simulink model "BoostPFC"  (R2024b)
settings: Solver=FixedStepAuto  StartTime=0.0  StopTime=3  FixedStep=Ts  RelTol=1e-3
PreLoadFcn:
  | BoostPFCData
values from neighbouring files (symbols this model uses):
  Delta = 1-V_I/V_O    (= 0.4)    [DCDCTuning.m]
  f_sw = 50e3    (= 50000)    [DCDCTuning.m]
  Ki_v = X_pid(2)    [DCDCTuning.m]
  Kp_v = X_pid(1)    [DCDCTuning.m]
  R = 40    [DCDCTuning.m]
  Ts = 1/(30*f_sw)    (= 6.66666666667e-07)    [DCDCTuning.m]
  Tsc = 1/(f_sw)    (= 2e-05)    [DCDCTuning.m]
  V_I = 24    [DCDCTuning.m]
undefined symbols (not defined in the file or in its folder): Ki_i, Kp_i
libraries: fl_lib x14, nesl_utility x7, eePwmGenerator x1, ee_lib x1, spsPowerLib x1
CloseFcn:
  | try,close(h1_ee_BoostPFC),end
  | clear h1_BoostPFC
  | 
  | clear simlog_BoostPFC
  | clear logsout_BoostPFC
Description:
  | Power Factor Correction for CCM Boost Converter
  | 
  | %
settings Model: Creator=The MathWorks, Inc.  LastModifiedBy=Will
settings SolverCC: AlgebraicLoopSolver=TrustRegion  MaxZcPerStep=1
settings DataIOCC: FinalStateName=xTransients  InitialState=xTransients  SaveOperatingPoint=on  SaveOutput=off  SignalLogging=off  DSMLogging=off  SaveTime=off  ReturnWorkspaceOutputs=off
settings OptimizationCC: ReuseModelBlockBuffer=off  LifeSpan=inf
settings DebuggingCC: UnconnectedInputMsg=warning  UnconnectedOutputMsg=warning  UnconnectedLineMsg=warning  SFUnexpectedBacktrackingDiag=warning  SFNoUnconditionalDefaultTransitionDiag=warning  SFExecutionAtInitializationDiag=none  ArithmeticOperatorsInVariantConditions=warning
settings ModelReferenceCC: EnableRefExpFcnMdlSchedulingChecks=on
settings SFSimCC: SimUseLocalCustomCode=off  CustomCodeUndefinedFunction=UseInterfaceOnly
settings RTWCC: RTWUseLocalCustomCode=off  GPUComputeCapability=3.5  DLArmComputeVersion=19.05
settings CodeAppCC: StateflowObjectComments=on
settings GRTTargetCC: TargetLangStandard=C89/C90 (ANSI)
settings ConfigComp: CovMetricSettings=dw  CovSaveCumulativeToWorkspaceVar=on  CovSaveSingleToWorkspaceVar=on  CovExternalEMLEnable=off
settings SimscapeCC: SimscapeNormalizeSystem=off  SimscapeLogType=local  SimscapeLogName=simlog_BoostPFC  SimscapeLogLimitData=off

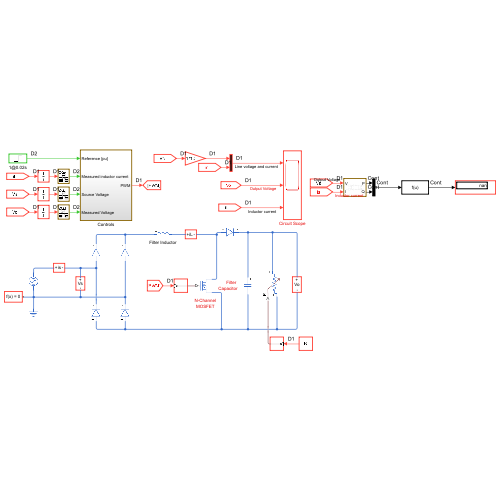
[thumbnail: Simulink's stored preview of the top-level diagram]
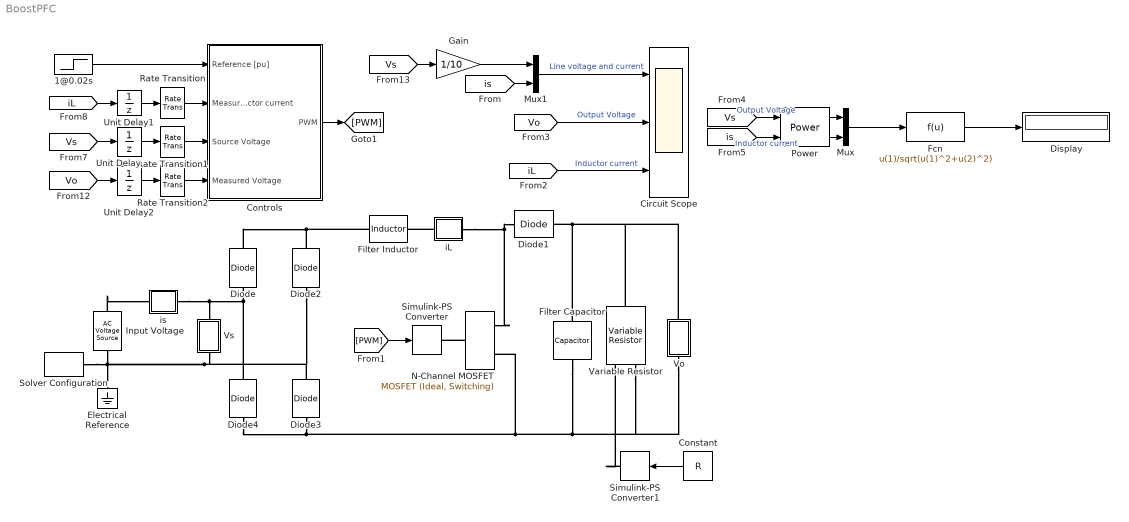
== system BoostPFC ==
  1@0.02s : Step  Time=0.02  After=40  SampleTime=Tsc
  Circuit Scope : Scope  NumInputPorts=3
  Constant : Constant  Value=R  SampleTime=Ts
  Controls : Subsystem
  Diode{,2..4} (4 alike) : fl_lib/Electrical/Electrical Elements/Diode  Vf=0.6 V  Ron=0.3 Ohm  Goff=1e-8 1/Ohm  i_specify=off  i_priority=None  i=0 A  i_nominal_specify=off  i_nominal_value=1  i_nominal_unit=A  v_specify=off  v_priority=None  v=0 V  v_nominal_specify=off  v_nominal_value=1  v_nominal_unit=V
  Diode1 : fl_lib/Electrical/Electrical Elements/Diode  Vf=0.55 V  Ron=0.36 Ohm  Goff=1e-8 1/Ohm  i_specify=off  i_priority=None  i=0 A  i_nominal_specify=off  i_nominal_value=1  i_nominal_unit=A  v_specify=off  v_priority=None  v=0 V  v_nominal_specify=off  v_nominal_value=1  v_nominal_unit=V
  Display : Display
  Electrical Reference : fl_lib/Electrical/Electrical Elements/Electrical Reference
  Fcn : Fcn  Expr=u(1)/sqrt(u(1)^2+u(2)^2)
  Filter Capacitor : fl_lib/Electrical/Electrical Elements/Capacitor  c=Cap F  r=r_C Ohm  g=0 1/Ohm  i_specify=off  i_priority=None  i=0 A  i_nominal_specify=off  i_nominal_value=1  i_nominal_unit=A  v_specify=off  v_priority=None  v=0 V  v_nominal_specify=off  v_nominal_value=1  v_nominal_unit=V  vc_specify=off  vc_priority=High  vc=0 V  vc_nominal_specify=off  vc_nominal_value=1  vc_nominal_unit=V
  Filter Inductor : fl_lib/Electrical/Electrical Elements/Inductor  l=L H  r=r_L Ohm  g=1e-9 1/Ohm  i_specify=off  i_priority=None  i=20 A  i_nominal_specify=off  i_nominal_value=1  i_nominal_unit=A  v_specify=off  v_priority=None  v=0 V  v_nominal_specify=off  v_nominal_value=1  v_nominal_unit=V  i_L_specify=off  i_L_priority=High  i_L=0 A  i_L_nominal_specify=off  i_L_nominal_value=1  i_L_nominal_unit=A
      settings: LogSimulationData=on
  Gain : Gain  Gain=1/10
  Input Voltage : fl_lib/Electrical/Electrical Sources/AC Voltage Source  amp=V_I*sqrt(2) V  shift=0 deg  frequency=f_line Hz
  Mux : Mux  Inputs=2
  Mux1 : Mux  Inputs=2
  N-Channel MOSFET : ee_lib/Semiconductors & Converters/MOSFET (Ideal, Switching)  port_option=ee.enum.controlport.ps  Rds=0.005 Ohm  Goff=1e-6 1/Ohm  Vth=0.5 V  diode_param=2  diode_Vf=0.88 V  diode_Ron=0.001 Ohm  diode_Goff=1e-5 1/Ohm  diode_C=5e-8 F  diode_iRM=-235 A  diode_iF=300 A  diode_idot=-50 A/us  diode_trr_param=1  diode_trr_factor=3  diode_trr=15 us  diode_Qrr=1.5e+3 s*uA  ids_specify=off  ids_priority=None  ids=0 A  ids_nominal_specify=off  ids_nominal_value=1  ids_nominal_unit=A  vds_specify=off  vds_priority=None  vds=0 V  vds_nominal_specify=off  vds_nominal_value=1  vds_nominal_unit=V  vgs_specify=off  vgs_priority=None  vgs=0 V  vgs_nominal_specify=off  vgs_nominal_value=1  vgs_nominal_unit=V  thermal_loss_option=ee.enum.converters.thermalLossOption.constantvalues  Von_data=[0, 1.8, 3.2, 6, 10, 16; 0, 2, 5.5, 9.5, 15, 25] V  Tj=[298.15, 448.15] K  Iout_data=[0, 20, 40, 60, 80, 100] A  Eon_data=[0, 55.04, 124.57, 235.53, 362.12; 0, 71.25, 161.25, 304.88, 468.75] * 1e-6 J  Eoff_data=[0, 18, 30, 56.1, 76.5; 0, 22.5, 37.5, 70.13, 95.63] * 1e-6 J  Eon_data_3D=[zeros(2, 5, 3)] J  Eoff_data_3D=[zeros(2, 5, 3)] J  Tj_loss=[298.15, 448.15] K  Iout_data_loss=[0, 10, 20, 30, 40] A  tabulateWithVds=false  Vds_loss=[0, 150, 300] V  Eon_scalar=22.86e-3 J  Eoff_scalar=17.14e-3 J  Voff=300 V  Iout_scalar=600 A  useCurrentFromPreviousCycle=false  useVoltageFromPreviousCycle=false  diodeModelType=ee.enum.converters.diodeModelType.pwl  diodeTableType=ee.enum.diode.tableType.IfMat  diode_ReverseIVType=ee.enum.diode.diodeReverseIV.constant  diode_IfMat=[.07, .12, .19, 1.75, 4.24, 7.32, 11.2; .16, .3, .72, 2.14, 4.02, 6.35, 9.12] A  diode_VfMat=[.9, 1.15, 1.25, 1.5, 1.75, 2.17, 2.6, 2.85; .58, .68, .75, 1.1, 1.38, 1.77, 2.27, 2.7] V  diode_TjVec=[25, 125] degC  diode_VfVec=[.5, .7, .9, 1.3, 1.7, 2.1, 2.5] V  diode_IfVec=[.1, .2, .5, 1, 2, 4, 7, 10] A  diode_IrMat=[1e-06, 2e-06, 5e-06, 1e-05, 2.5e-05, 5e-05, .0001; 2e-06, 5e-06, 1e-05, 4e-05, 8e-05, .0002, .0005] A  diode_VrMat=[10, 100, 200, 250, 300, 325, 350; 10, 70, 160, 220, 270, 300, 320] V  diode_VrVec=[10, 20, 40, 50, 70, 80, 100] V  diode_IrVec=[1e-06, 2e-06, 5e-06, 1e-05, 2e-05, 5e-05, .0001] A  diode_Vr=-600 V  diode_Ls=150 nH  diode_Erec=0.03 J  diode_rec_loss_model=ee.enum.diode.reverseRecoveryModel.fixed  diode_ErecVal=0 J  diode_scaleWithIandV=true  diode_ErecMat=zeros(2, 3) J  diode_TjrecVec=[298.15, 398.15] K  diode_IfrecVec=[.1, 1, 10] A  diode_IrecVal=10 A  diode_VrecVal=10 V  diode_tFilter=1 / 1000 / 100 s  separateThermalPortForDiode=false  thermal_network_parameterization=ee.enum.thermalNetworkTopology.external  Rth=[.03, .2] K/W  Rth_Cauer=[.03, .1, .2] K/W  Rth_Foster=[.03, .2] K/W  thermal_mass_parameterization=ee.enum.thermalNetwork.timeconstant  thermal_mass=[3, 25] J/K  thermal_mass_Cauer=[3, 10, 25] J/K  thermal_mass_Foster=[33, 50] J/K  thermal_time_constant=[.1, 5] s  thermal_time_constant_Cauer=[.1, 1, 5] s  thermal_time_constant_Foster=[1, 10] s  thermal_mass_initial_temperatures=[25, 25] degC  thermal_mass_initial_temperatures_Cauer=[25, 25, 25] degC  junction_thermal_mass=0.1 J/K  Tvec_initial_Foster=[25, 25, 25, 25] degC  RthDiode=[.03, .2] K/W  RthCauerDiode=[.03, .1, .2] K/W  RthFosterDiode=[.03, .2] K/W  thermalMassDiode=[3, 25] J/K  thermalMassCauerDiode=[3, 10, 25] J/K  thermalMassFosterDiode=[33, 50] J/K  thermalTauDiode=[.1, 5] s  thermalTauCauerDiode=[.1, 1, 5] s  thermalTauFosterDiode=[1, 10] s  thermalMassInitTempDiode=[25, 25] degC  thermalMassInitTempCauerDiode=[25, 25, 25] degC  junctionthermalMassDiode=0.1 J/K  TVecInitialFosterDiode=[25, 25, 25, 25] degC  no_thermal_network=0  mosfet_junction_temperature_specify=off  mosfet_junction_temperature_priority=None  mosfet_junction_temperature=25 degC  mosfet_junction_temperature_nominal_specify=off  mosfet_junction_temperature_nominal_value=1  mosfet_junction_temperature_nominal_unit=degC  diode_junction_temperature_specify=off  diode_junction_temperature_priority=None  diode_junction_temperature=25 degC  diode_junction_temperature_nominal_specify=off  diode_junction_temperature_nominal_value=1  diode_junction_temperature_nominal_unit=degC  Qj_specify=off  Qj_priority=None  Qj=0 W  Qj_nominal_specify=off  Qj_nominal_value=1  Qj_nominal_unit=W  accumulatedSwitchingLosses_specify=off  accumulatedSwitchingLosses_priority=None  accumulatedSwitchingLosses=0 J
  Power : spsPowerLib/Power  Freq=60  Vinit=[1, 0]  Iinit=[1, 0]  Ts=0
  Rate Transition : RateTransition  OutPortSampleTime=Tsc
  Rate Transition1 : RateTransition  OutPortSampleTime=Tsc
  Rate Transition2 : RateTransition  OutPortSampleTime=Tsc
  Simulink-PS Converter : nesl_utility/Simulink-PS Converter  PhysicalDomain=network_engine_domain  SubClassName=ps_input  LeftPortType=input  RightPortType=output  PseudoPeriodic=off  Frequencies=[]  NoiseDistribution=none  NoiseParameters=[]  Unit=1  AffineConversion=off  FilteringAndDerivatives=provide  SimscapeFilterOrder=1  InputFilterTimeConstant=0.001  UdotUserProvided=0
  Simulink-PS Converter1 : nesl_utility/Simulink-PS Converter  PhysicalDomain=network_engine_domain  SubClassName=ps_input  LeftPortType=input  RightPortType=output  PseudoPeriodic=off  Frequencies=[]  NoiseDistribution=none  NoiseParameters=[]  Unit=1  AffineConversion=off  FilteringAndDerivatives=provide  SimscapeFilterOrder=1  InputFilterTimeConstant=0.001  UdotUserProvided=0
  Solver Configuration : nesl_utility/Solver Configuration  PhysicalDomain=network_engine_domain  SubClassName=solver  LeftPortType=input  RightPortType=generic  Tones=[]  Harmonics=[]  SimulateNoise=off  Profile=off  UseLocalSampling=off  EnableSwitchedLinearOptims=on  FrequencyDomain=off  UseCCode=off  RelTol=0.001  AbsTol=1e-06  MinStep=1e-09  ToWorkspace=off  RevertToSquareIcSolve=off  NumHomotopyIterations=100  PhasorMode=off  PhasorModeNumHarmonics=1  ConsistencySolver=NEWTON_FTOL  IndexReductionMethod=DerivativeReplacement  DoDC=off  ResidualTolerance=1e-09  ConsistencyTolSource=GLOBAL  ConsistencyAbsTol=0.001  ConsistencyRelTol=0.001  ConsistencyTolFactor=0.001  UseLocalSolver=on  LocalSolverChoice=NE_BACKWARD_EULER_ADVANCER  ResolveIndetEquations=on  FunctionEvalNumThread=1  LocalSolverSampleTime=Ts  DoFixedCost=on  MaxNonlinIter=4  MaxModeIter=2  ComputeImpulses=off  ImpulseIterations=1  LinearAlgebra=auto  LinearAlgebraNumThread=0  EquationFormulation=NE_TIME_EF  DelaysMemoryBudget=1024  AutomaticFiltering=on  FilteringTimeConstant=0.001  PartitionStorageMethod=AS_NEEDED  PartitionMemoryBudget=1024  PartitionMethod=FAST  MultibodyUseLocalSolver=off  MultibodyLocalSolverChoice=ODE1  MultibodyLocalSolverSampleTime=0.001
  Unit Delay : UnitDelay  SampleTime=-1  HasFrameUpgradeWarning=on
  Unit Delay1 : UnitDelay  SampleTime=-1  HasFrameUpgradeWarning=on
  Unit Delay2 : UnitDelay  SampleTime=-1  HasFrameUpgradeWarning=on
  Variable Resistor : fl_lib/Electrical/Electrical Elements/Variable Resistor  Rmin=0 Ohm  thermalEnable=false  thermal_mass=1 J/K  i_specify=off  i_priority=None  i=0 A  i_nominal_specify=off  i_nominal_value=1  i_nominal_unit=A  v_specify=off  v_priority=None  v=0 V  v_nominal_specify=off  v_nominal_value=1  v_nominal_unit=V  T_specify=off  T_priority=None  T=300 K  T_nominal_specify=off  T_nominal_value=1  T_nominal_unit=K
  Vo : Subsystem
      mask Display:
      | disp('Vo')
      | port_label('Lconn',1,'+')
      | port_label('Rconn',1,'-')
  Vs : Subsystem
      mask Display:
      | disp('Vs')
      | port_label('Lconn',1,'+')
      | port_label('Rconn',1,'-')
  iL : Subsystem
      mask Display:
      | disp('iL')
      | port_label('Lconn',1,'+')
      | port_label('Rconn',1,'-')
  is : Subsystem
      mask Display:
      | disp('is')
      | port_label('Lconn',1,'+')
      | port_label('Rconn',1,'-')
  wires:
  [iL] -> Circuit Scope/3  "Inductor current"
  [Vs] -> Unit Delay/1
  Rate Transition/1 -> Controls/2(Measured inductor current)
  Unit Delay/1 -> Rate Transition1/1
  Unit Delay1/1 -> Rate Transition/1
  Unit Delay2/1 -> Rate Transition2/1
  [iL] -> Unit Delay1/1
  [Vo] -> Unit Delay2/1
  [is] -> Mux1/2
  [Vs] -> Gain/1
  Mux1/1 -> Circuit Scope/1  "Line voltage and current"
  [Vo] -> Circuit Scope/2  "Output Voltage"
  Gain/1 -> Mux1/1
  Rate Transition1/1 -> Controls/3(Source Voltage)
  Controls/1(PWM) -> [PWM]
  [PWM] -> Simulink-PS Converter/1
  Rate Transition2/1 -> Controls/4(Measured Voltage)
  Constant/1 -> Simulink-PS Converter1/1
  1@0.02s/1 -> Controls/1(Reference [pu])
  [Vs] -> Power/1  "Output Voltage"
  [is] -> Power/2  "Inductor current"
  Power/1 -> Mux/1
  Power/2 -> Mux/2
  Mux/1 -> Fcn/1
  Fcn/1 -> Display/1
  connections:
  N-Channel MOSFET/LConn1 -- Simulink-PS Converter/RConn1
  Filter Capacitor/LConn1 -- Variable Resistor/RConn1 -- Vo/LConn1 -- Diode1/RConn1
  Input Voltage/LConn1 -- is/LConn1
  iL/LConn1 -- Filter Inductor/RConn1
  N-Channel MOSFET/RConn1 -- iL/RConn1 -- Diode1/LConn1
  Simulink-PS Converter1/RConn1 -- Variable Resistor/LConn1
  Filter Inductor/LConn1 -- Diode/RConn1 -- Diode2/RConn1
  Vo/RConn1 -- Variable Resistor/LConn2 -- Filter Capacitor/RConn1 -- Diode4/LConn1 -- Diode3/LConn1 -- N-Channel MOSFET/RConn2
  is/RConn1 -- Diode/LConn1 -- Diode4/RConn1 -- Vs/LConn1
  Input Voltage/RConn1 -- Vs/RConn1 -- Diode2/LConn1 -- Diode3/RConn1 -- Solver Configuration/RConn1 -- Electrical Reference/LConn1

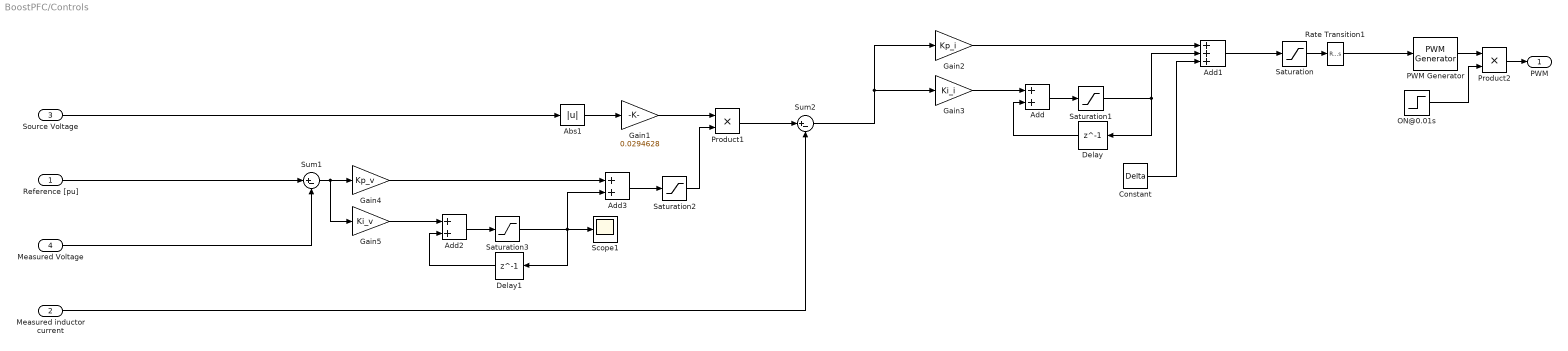
== system BoostPFC/Controls ==
  Reference [pu] : Inport
  Measured inductor current : Inport  Port=2
  Source Voltage : Inport  Port=3
  Measured Voltage : Inport  Port=4
  Abs1 : Abs  SaturateOnIntegerOverflow=off
  Add : Sum
  Add1 : Sum  Inputs=+++
  Add2 : Sum
  Add3 : Sum
  Constant : Constant  Value=Delta
  Delay : Delay  DelayLength=1  SampleTime=Tsc
  Delay1 : Delay  DelayLength=1  SampleTime=Tsc
  Gain1 : Gain  Gain=0.0294628
  Gain2 : Gain  Gain=Kp_i
  Gain3 : Gain  Gain=Ki_i
  Gain4 : Gain  Gain=Kp_v
  Gain5 : Gain  Gain=Ki_v
  ON@0.01s : Step  Time=0.01  SampleTime=Ts
  PWM Generator : eePwmGenerator/PWM Generator  CarrCount=Up  Tper=1/f_sw  Tdelay=0  Ts=Ts
  Product1 : Product
  Product2 : Product
  Rate Transition1 : RateTransition  OutPortSampleTime=Ts
  Saturation : Saturate  UpperLimit=0.99  LowerLimit=0.01
  Saturation1 : Saturate  UpperLimit=100  LowerLimit=-100
  Saturation2 : Saturate  UpperLimit=4  LowerLimit=0
  Saturation3 : Saturate  UpperLimit=4  LowerLimit=-4
  Scope1 : Scope
  Sum1 : Sum  Inputs=|+-
  Sum2 : Sum  Inputs=|+-
  PWM : Outport  VectorParamsAs1DForOutWhenUnconnected=off
  wires:
  Measured Voltage/1 -> Sum1/2
  Measured inductor current/1 -> Sum2/2
  ON@0.01s/1 -> Product2/2
  Product2/1 -> PWM/1
  PWM Generator/1 -> Product2/1
  Reference [pu]/1 -> Sum1/1
  Source Voltage/1 -> Abs1/1
  Abs1/1 -> Gain1/1
  Sum2/1 -> Gain2/1, Gain3/1
  Gain3/1 -> Add/1
  Add/1 -> Saturation1/1
  Gain2/1 -> Add1/1
  Delay/1 -> Add/2
  Constant/1 -> Add1/3
  Saturation1/1 -> Add1/2, Delay/1
  Rate Transition1/1 -> PWM Generator/1
  Saturation/1 -> Rate Transition1/1
  Add3/1 -> Saturation2/1
  Saturation3/1 -> Scope1/1, Add3/2, Delay1/1
  Gain4/1 -> Add3/1
  Delay1/1 -> Add2/2
  Add2/1 -> Saturation3/1
  Gain5/1 -> Add2/1
  Sum1/1 -> Gain5/1, Gain4/1
  Gain1/1 -> Product1/1
  Saturation2/1 -> Product1/2
  Product1/1 -> Sum2/1
  Add1/1 -> Saturation/1

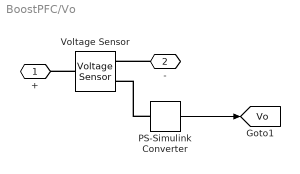
== system BoostPFC/Vo ==
  PS-Simulink Converter : nesl_utility/PS-Simulink Converter  PhysicalDomain=network_engine_domain  SubClassName=ps_output  LeftPortType=input  RightPortType=output  PseudoPeriodic=off  Frequencies=[]  VectorFormat=1-D array  Unit=1  AffineConversion=off
  Voltage Sensor : fl_lib/Electrical/Electrical Sensors/Voltage Sensor
      settings: LogSimulationData=on
  + : PMIOPort  Side=Left
  - : PMIOPort  Port=2  Side=Right
  tag scope: Vo=global
  wires:
  PS-Simulink Converter/1 -> [Vo]
  connections:
  PS-Simulink Converter/LConn1 -- Voltage Sensor/RConn1
  Voltage Sensor/LConn1 -- +/RConn1
  -/RConn1 -- Voltage Sensor/RConn2

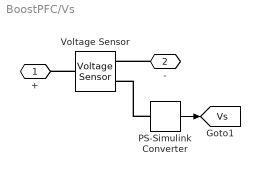
== system BoostPFC/Vs ==
  PS-Simulink Converter : nesl_utility/PS-Simulink Converter  PhysicalDomain=network_engine_domain  SubClassName=ps_output  LeftPortType=input  RightPortType=output  PseudoPeriodic=off  Frequencies=[]  VectorFormat=1-D array  Unit=1  AffineConversion=off
  Voltage Sensor : fl_lib/Electrical/Electrical Sensors/Voltage Sensor
      settings: LogSimulationData=on
  + : PMIOPort  Side=Left
  - : PMIOPort  Port=2  Side=Right
  tag scope: Vs=global
  wires:
  PS-Simulink Converter/1 -> [Vs]
  connections:
  -/RConn1 -- Voltage Sensor/RConn2
  Voltage Sensor/LConn1 -- +/RConn1
  PS-Simulink Converter/LConn1 -- Voltage Sensor/RConn1

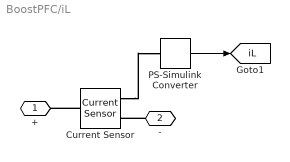
== system BoostPFC/iL ==
  Current Sensor : fl_lib/Electrical/Electrical Sensors/Current Sensor
  PS-Simulink Converter : nesl_utility/PS-Simulink Converter  PhysicalDomain=network_engine_domain  SubClassName=ps_output  LeftPortType=input  RightPortType=output  PseudoPeriodic=off  Frequencies=[]  VectorFormat=1-D array  Unit=1  AffineConversion=off
  + : PMIOPort  Side=Left
  - : PMIOPort  Port=2  Side=Right
  tag scope: iL=global
  wires:
  PS-Simulink Converter/1 -> [iL]
  connections:
  Current Sensor/LConn1 -- +/RConn1
  Current Sensor/RConn1 -- PS-Simulink Converter/LConn1
  -/RConn1 -- Current Sensor/RConn2

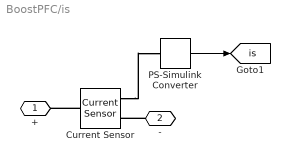
== system BoostPFC/is ==
  Current Sensor : fl_lib/Electrical/Electrical Sensors/Current Sensor
      settings: LogSimulationData=on
  PS-Simulink Converter : nesl_utility/PS-Simulink Converter  PhysicalDomain=network_engine_domain  SubClassName=ps_output  LeftPortType=input  RightPortType=output  PseudoPeriodic=off  Frequencies=[]  VectorFormat=1-D array  Unit=1  AffineConversion=off
  + : PMIOPort  Side=Left
  - : PMIOPort  Port=2  Side=Right
  tag scope: is=global
  wires:
  PS-Simulink Converter/1 -> [is]
  connections:
  -/RConn1 -- Current Sensor/RConn2
  Current Sensor/RConn1 -- PS-Simulink Converter/LConn1
  Current Sensor/LConn1 -- +/RConn1
